simulink model "practica6"  (R2019b)
settings: Solver=FixedStepAuto  StartTime=0.0  StopTime=10.0  RelTol=1e-3  EnableMultiTasking=on
undefined symbols (not defined in the file or in its folder): Boton, Ciclo, Color, Estados, US
libraries: legoev3lib x11
settings Model: ExtModeTrigDuration=2  Creator=alumnopr13  LastModifiedBy=alumnopr13
settings SolverCC: PositivePriorityOrder=on
settings OptimizationCC: EnhancedBackFolding=on  PassReuseOutputArgsAs=Individual arguments  ZeroExternalMemoryAtStartup=off  ZeroInternalMemoryAtStartup=off  MaxStackSize=64  OptimizeBlockOrder=speed  DifferentSizesBufferReuse=on  OptimizationCustomize=off  EfficientTunableParamExpr=on
settings DebuggingCC: ParameterTunabilityLossMsg=error
settings HardwareCC: ProdBitPerPointer=32  ProdBitPerSizeT=32  ProdBitPerPtrDiffT=32  ProdLargestAtomicInteger=Long  ProdWordSize=32  ProdHWDeviceType=ARM Compatible->ARM 9
settings SFSimCC: MATLABDynamicMemAlloc=off
settings RTWCC: SystemTargetFile=ert.tlc  HardwareBoard=LEGO MINDSTORMS EV3  TLCOptions="-aInlineSetEventsForThisBaseRateFcn=TLC_FALSE -aSuppressMultiTaskScheduler=TLC_FALSE  -aRateBasedStepFcn=0"  TemplateMakefile=ert_default_tmf  GenerateReport=on  Toolchain=Sourcery G++ Lite v2009q3  IncludeHyperlinkInReport=on  LaunchReport=on  GenerateTraceInfo=on  GenerateTraceReport=on  GenerateTraceReportSl=on  GenerateTraceReportSf=on  GenerateTraceReportEml=on
settings CodeAppCC: ForceParamTrailComments=on  IgnoreCustomStorageClasses=off  OperatorAnnotations=on  SimulinkDataObjDesc=on  SFDataObjDesc=on  InsertBlockDesc=on
settings ERTTargetCC: SupportContinuousTime=on  SupportVariableSizeSignals=on

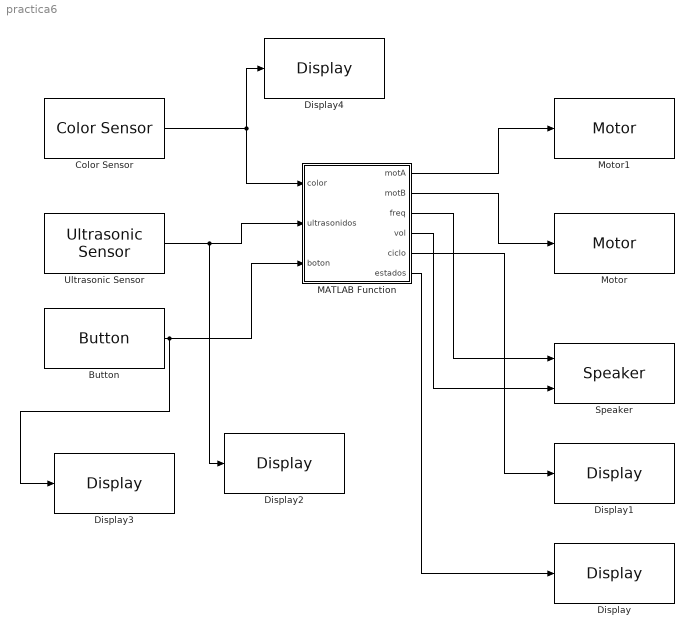
== system practica6 ==
  Button : legoev3lib/Button  buttonType=Down  sampleTime=0.1
      settings: SourceProductName=Simulink Support Package for LEGO MINDSTORMS EV3 Hardware  SourceProductBaseCode=LEGOEV3
  Color Sensor : legoev3lib/Color Sensor  portNumber=4  mode=Color  sampleTime=0.1
      settings: SourceProductName=Simulink Support Package for LEGO MINDSTORMS EV3 Hardware  SourceProductBaseCode=LEGOEV3
  Display : legoev3lib/Display  slcdStr=Estados:  slcdLine=3  slcdFormat=Decimal
      settings: SourceProductName=Simulink Support Package for LEGO MINDSTORMS EV3 Hardware  SourceProductBaseCode=LEGOEV3
  Display1 : legoev3lib/Display  slcdStr=Ciclo:  slcdLine=2  slcdFormat=Decimal
      settings: SourceProductName=Simulink Support Package for LEGO MINDSTORMS EV3 Hardware  SourceProductBaseCode=LEGOEV3
  Display2 : legoev3lib/Display  slcdStr=US:  slcdLine=1  slcdFormat=Decimal
      settings: SourceProductName=Simulink Support Package for LEGO MINDSTORMS EV3 Hardware  SourceProductBaseCode=LEGOEV3
  Display3 : legoev3lib/Display  slcdStr=Boton:  slcdLine=4  slcdFormat=Decimal
      settings: SourceProductName=Simulink Support Package for LEGO MINDSTORMS EV3 Hardware  SourceProductBaseCode=LEGOEV3
  Display4 : legoev3lib/Display  slcdStr=Color:  slcdLine=5  slcdFormat=Decimal
      settings: SourceProductName=Simulink Support Package for LEGO MINDSTORMS EV3 Hardware  SourceProductBaseCode=LEGOEV3
  MATLAB Function : MATLAB Function  TreatAsAtomicUnit=on
  Motor : legoev3lib/Motor  sportNumber=D  sstopAction=Brake
  Motor1 : legoev3lib/Motor  sportNumber=A  sstopAction=Brake
  Speaker : legoev3lib/Speaker  sinputMode=Frequency and volume  sspeakerFreq=100  sspeakerVolume=50  sspeakerDuration=1000
      settings: SourceProductName=Simulink Support Package for LEGO MINDSTORMS EV3 Hardware  SourceProductBaseCode=LEGOEV3
  Ultrasonic Sensor : legoev3lib/Ultrasonic Sensor  PortNumber=1  sampleTime=0.1
      settings: SourceProductName=Simulink Support Package for LEGO MINDSTORMS EV3 Hardware  SourceProductBaseCode=LEGOEV3
  wires:
  Color Sensor/1 -> Display4/1, MATLAB Function/1(color)
  Ultrasonic Sensor/1 -> Display2/1, MATLAB Function/2(ultrasonidos)
  Button/1 -> Display3/1, MATLAB Function/3(boton)
  MATLAB Function/1(motA) -> Motor1/1
  MATLAB Function/2(motB) -> Motor/1
  MATLAB Function/3(freq) -> Speaker/1
  MATLAB Function/4(vol) -> Speaker/2
  MATLAB Function/5(ciclo) -> Display1/1
  MATLAB Function/6(estados) -> Display/1

== matlab function practica6/MATLAB Function ==
  data: color input; ultrasonidos input; motA output; motB output; freq output; vol output; boton input; ciclo output; estados output
function [motA, motB, freq, vol, ciclo, estados]= Planner(color, ultrasonidos, boton)
    persistent ciclos
    persistent pA
    persistent pB
    persistent comido
    persistent avoid
    
    if isempty(ciclos)
       ciclos=50;
    end
    if isempty(pA)
       pA=0;
    end
    if isempty(pB)
       pB=0;
    end
    if isempty(comido)
       comido=false;
    end
    if isempty(avoid)
       avoid = false;
    end
    freq = 0;
    vol = 0;
    if(comido && boton==1)
        freq = 0;
        vol = 0;
        motA = pA;
        motB = pB;
        comido = false;
        avoid = false;
    elseif(not(comido))    
        if(color==6)
            foraging();
        elseif(ultrasonidos<=30 || avoid)
            obstacle_avoid();
        else
            wander();
        end
    else
        motA = 0;
        motB = 0;
    end
    
    ciclo = ciclos;
    if(comido)
        estados = 2;
    elseif(avoid)
        estados = 1;
    else
        estados = 0;
    end
    
    function [] = wander()
        if(ciclos==50)
            motA=randi([0,50]);
            pA = motA;
            motB=randi([0,50]);
            pB = motB;
            ciclos = 1;
        else
            motA = pA;
            motB = pB;
            ciclos = ciclos+1;
        end
    end

    function [] = obstacle_avoid()
        if(ultrasonidos<=40)
            motA = -20;
            motB = -20;
            avoid = true;
        else
            motA=40;
            motB=5;
            pA=40;
            pB=5;
            ciclos=45;
            avoid = false;
        end
    end

    function [] = foraging()
            motA=0;
            motB=0;
            pA=0;
            pB=0;
            freq=100;
            vol = 10;
            comido = true;
    end
end
